simulink model "Punto1_522"  (R2019a)
settings: Solver=VariableStepAuto  StartTime=0.0  StopTime=3  MaxStep=1e-4  RelTol=1e-3
values from neighbouring files (symbols this model uses):
  alfa_cu = 3.9 * 10^(-3)    (= 0.0039)    [Datos.m]
  bl = 0    [Datos.m]
  bm = 1.5 * 10^(-5)    (= 1.5e-05)    [Datos.m]
  Cts = 0.818    [Datos.m]
  Id0 = 0    [Datos.m]    (also in punto6plot.m = 0.5)
  Jl = 0.2520    (= 0.252)    [Datos.m]
  Jm = 3.1 * 10^(-6)    (= 3.1e-06)    [Datos.m]
  Ki0 = 5000*Lls    (= 4)    [Datos.m]
  Kid = 5000*Ld    (= 33)    [Datos.m]
  Kiq = 5000*Lq    (= 29)    [Datos.m]
  lambda_m_r = 0.01546    [Datos.m]
  Ld = 6.6e-3    (= 0.0066)    [Datos.m]
  Lq = 5.8e-3    (= 0.0058)    [Datos.m]
  Pp = 3    [Datos.m]
  r = 314.3008    [Datos.m]
  Rts_amb = 146.7    [Datos.m]
undefined symbols (not defined in the file or in its folder): magnitude
settings Model: Creator=renzo  LastModifiedBy=renzo

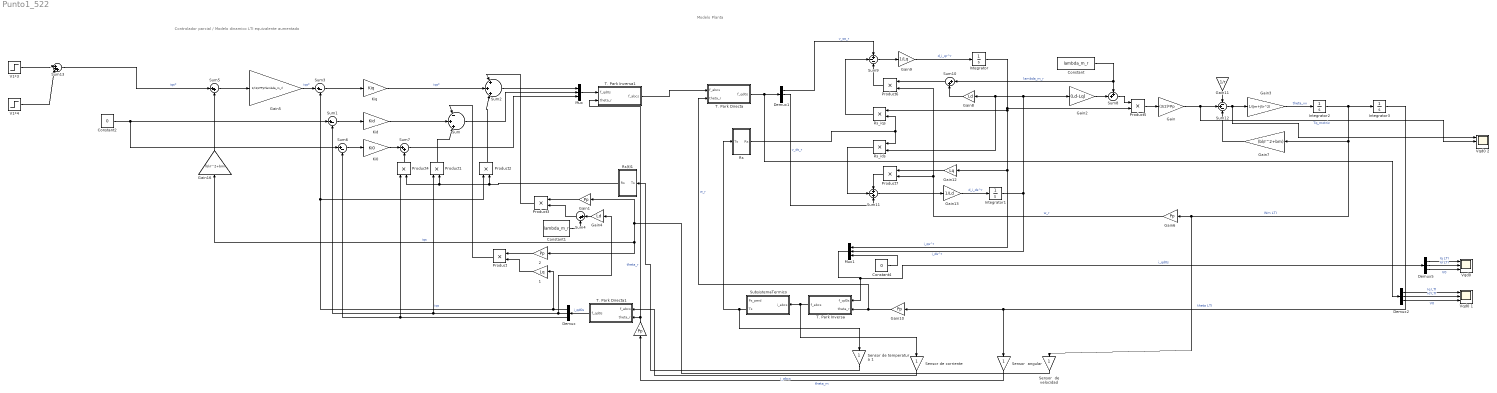
== system Punto1_522 ==
  note: Controlador parcial / Modelo dinamico LTI equivalente aumentado
  note: Modelo Planta
  " " : Gain  Gain=Pp
  " 1" : Gain  Gain=Lq
  " 2" : Gain  Gain=Pp
  Constant : Constant  Value=lambda_m_r
  Constant1 : Constant  Value=lambda_m_r
  Constant2 : Constant  Value=0
  Constant4 : Constant  Value=0
  Demux{,1..2,5} (4 alike) : Demux  Outputs=3
  Gain : Gain  Gain=(3/2)*Pp
  Gain1 : Gain  Gain=Pp
  Gain10 : Gain  Gain=Pp
  Gain11 : Gain  Gain=1/r
  Gain12 : Gain  Gain=Lq
  Gain13 : Gain  Gain=1/Ld
  Gain16 : Gain  Gain=(bl/r^2+bm)
  Gain2 : Gain  Gain=(Ld-Lq)
  Gain3 : Gain  Gain=1/(Jm+Jl/r^2)
  Gain4 : Gain  Gain=Ld
  Gain5 : Gain  Gain=1/(3/2*Pp*lambda_m_r)
  Gain6 : Gain  Gain=Pp
  Gain7 : Gain  Gain=(bl/r^2+bm)
  Gain8 : Gain  Gain=Ld
  Gain9 : Gain  Gain=1/Lq
  Integrator : Integrator
  Integrator1 : Integrator  InitialCondition=Id0
  Integrator2 : Integrator
  Integrator3 : Integrator
  Ki0 : Gain  Gain=Ki0
  Kid : Gain  Gain=Kid
  Kiq : Gain  Gain=Kiq
  Mux : Mux  Inputs=3
  Mux1 : Mux  Inputs=3
  Product{,1..7} (8 alike) : Product
  Rs : Subsystem
  Rs(t)1 : Subsystem
  Rs_ids : Product
  Rs_iqs : Product
  Sensor  angular : Gain
  Sensor  de velocidad : Gain
  "Sensor de corriente " : Gain
  Sensor de temperatura 1 : Gain
  SubsistemaTermico : Subsystem
  Sum : Sum  Inputs=|-|+|+|
  Sum1 : Sum  Inputs=|+-
  Sum{4..5,7,10} (4 alike) : Sum  Inputs=|++
  Sum11 : Sum  Inputs=+-+
  Sum12 : Sum  Inputs=-+-
  Sum13 : Sum  Inputs=|+++
  Sum2 : Sum  Inputs=|+|+|+|
  Sum3 : Sum  Inputs=|+-
  Sum6 : Sum  Inputs=|+-
  Sum8 : Sum  Inputs=++|
  Sum9 : Sum  Inputs=+--
  T. Park Directa : Subsystem
  T. Park Directa1 : Subsystem
  T. Park Inversa : Subsystem
  T. Park Inversa1 : Subsystem
  V1*3 : Step  Time=0.1  After=0.1  SampleTime=0
  V1*4 : Step  Time=0.2  After=-0.1  SampleTime=0
  "Vqd0 " : Scope  NumInputPorts=3
  Vqd0 1 : Scope  NumInputPorts=3
  Vqd0 2 : Scope  NumInputPorts=3
  wires:
  Gain16/1 -> Sum5/2
  Sum1/1 -> Kid/1
  Gain5/1 -> Sum3/1  "iqs*"
  Constant2/1 -> Sum6/1, Sum1/1
  Sum7/1 -> Mux/3
  Demux/1 -> " 1"/1, Sum3/2, Product2/1  "iqs"
  Sum4/1 -> Product3/2
  Sensor de temperatura 1/1 -> Rs(t)1/1(Ts)
  Ki0/1 -> Sum7/1
  Constant1/1 -> Sum4/2
  Sum6/1 -> Ki0/1
  Product4/1 -> Sum7/2
  Product3/1 -> Sum2/1
  Demux/3 -> Product4/1, Sum6/2
  Sum3/1 -> Kiq/1
  Rs(t)1/1(Rs) -> Product4/2, Product1/2, Product2/2
  Sum5/1 -> Gain5/1
  " 2"/1 -> Product/1
  " 1"/1 -> Product/2
  Kiq/1 -> Sum2/2  "iqs*"
  Gain1/1 -> Product3/1
  Sum/1 -> Mux/2
  Gain4/1 -> Sum4/1
  Product1/1 -> Sum/3
  Sum2/1 -> Mux/1
  Product/1 -> Sum/1
  Sensor  de velocidad/1 -> Gain16/1, " 2"/1, Gain1/1  "iqs"
  Mux/1 -> T. Park Inversa1/1(f_qd0s)
  " "/1 -> T. Park Inversa1/2(theta_r), T. Park Directa1/2(theta_r)  "theta_r"
  Kid/1 -> Sum/2
  Sensor  angular/1 -> " "/1  "theta_m"
  "Sensor de corriente "/1 -> T. Park Directa1/1(f_abcs)  "i_abcs"
  T. Park Directa1/1(f_qd0s) -> Demux/1  "i_qd0s"
  Product2/1 -> Sum2/3
  T. Park Inversa1/1(f_abcs) -> T. Park Directa/1(f_abcs)
  Demux/2 -> Gain4/1, Sum1/2, Product1/1
  Sum8/1 -> Product5/1
  T. Park Directa/1(f_qd0s) -> Demux2/1, Demux1/1
  Gain13/1 -> Integrator1/1  "d_i_ds^r"
  Rs_iqs/1 -> Sum9/2
  Gain2/1 -> Sum8/2
  T. Park Inversa/1(f_abcs) -> "Sensor de corriente "/1, SubsistemaTermico/1(i_abcs)
  Gain8/1 -> Sum10/2
  Product7/1 -> Sum11/1
  Sum10/1 -> Product6/1
  Gain7/1 -> Sum12/3
  Gain/1 -> Vqd0 2/2, Sum12/2  "Tq_motriz"
  Integrator3/1 -> Sensor  angular/1, Gain10/1  "theta LTI"
  Sum12/1 -> Vqd0 2/1, Gain3/1
  Rs_ids/1 -> Sum11/2
  Gain10/1 -> T. Park Directa/2(theta_r), T. Park Inversa/2(theta_r)  "w_r"
  Rs/1(Rs) -> Rs_ids/1, Rs_iqs/2
  Constant4/1 -> Mux1/3
  SubsistemaTermico/2(Ts) -> Sensor de temperatura 1/1, Rs/1(Ts)
  Mux1/1 -> Demux5/1, T. Park Inversa/1(f_qd0s)  "i_qd0s"
  Gain3/1 -> Integrator2/1  "theta_vv"
  Integrator/1 -> Product5/2, Mux1/1, Gain12/1, Rs_iqs/1  "i_qs^r"
  Sum11/1 -> Gain13/1
  Product5/1 -> Gain/1
  Integrator1/1 -> Gain8/1, Rs_ids/2, Gain2/1, Mux1/2  "i_ds^r"
  Gain9/1 -> Integrator/1  "d_i_qr^r"
  Integrator2/1 -> Sensor  de velocidad/1, Gain6/1, Gain7/1, Integrator3/1  "Wm LTI"
  Product6/1 -> Sum9/3
  Gain6/1 -> Product6/2, Product7/2  "w_r"
  Demux1/1 -> Sum9/1  "v_qs_r"
  Demux1/2 -> Sum11/3  "v_ds_r"
  Gain11/1 -> Sum12/1
  Sum9/1 -> Gain9/1
  Constant/1 -> Sum8/1, Sum10/1  "lambda_m_r"
  Gain12/1 -> Product7/1
  Demux5/1 -> "Vqd0 "/1  "Iq LTI"
  Demux5/2 -> "Vqd0 "/2  "Id LTI"
  Demux5/3 -> "Vqd0 "/3  "V0"
  Demux2/1 -> Vqd0 1/1  "Iq LTI"
  Demux2/2 -> Vqd0 1/2  "Id LTI"
  Demux2/3 -> Vqd0 1/3  "V0"
  V1*4/1 -> Sum13/2
  Sum13/1 -> Sum5/1  "iqs*"
  V1*3/1 -> Sum13/1

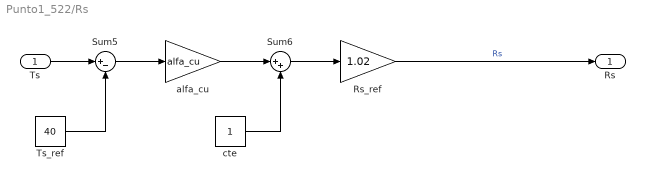
== system Punto1_522/Rs ==
  Ts : Inport
  Rs_ref : Gain  Gain=1.02
  Sum5 : Sum  Inputs=|+-
  Sum6 : Sum  Inputs=|++
  Ts_ref : Constant  Value=40
  alfa_cu : Gain  Gain=alfa_cu
  cte : Constant
  Rs : Outport
  wires:
  Ts_ref/1 -> Sum5/2
  Sum5/1 -> alfa_cu/1
  Sum6/1 -> Rs_ref/1
  Ts/1 -> Sum5/1
  alfa_cu/1 -> Sum6/1
  cte/1 -> Sum6/2
  Rs_ref/1 -> Rs/1  "Rs"

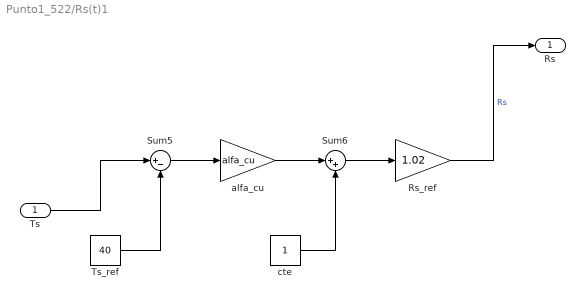
== system Punto1_522/Rs(t)1 ==
  Ts : Inport
  Rs_ref : Gain  Gain=1.02
  Sum5 : Sum  Inputs=|+-
  Sum6 : Sum  Inputs=|++
  Ts_ref : Constant  Value=40
  alfa_cu : Gain  Gain=alfa_cu
  cte : Constant
  Rs : Outport
  wires:
  alfa_cu/1 -> Sum6/1
  Sum6/1 -> Rs_ref/1
  Rs_ref/1 -> Rs/1  "Rs"
  Ts_ref/1 -> Sum5/2
  cte/1 -> Sum6/2
  Ts/1 -> Sum5/1
  Sum5/1 -> alfa_cu/1

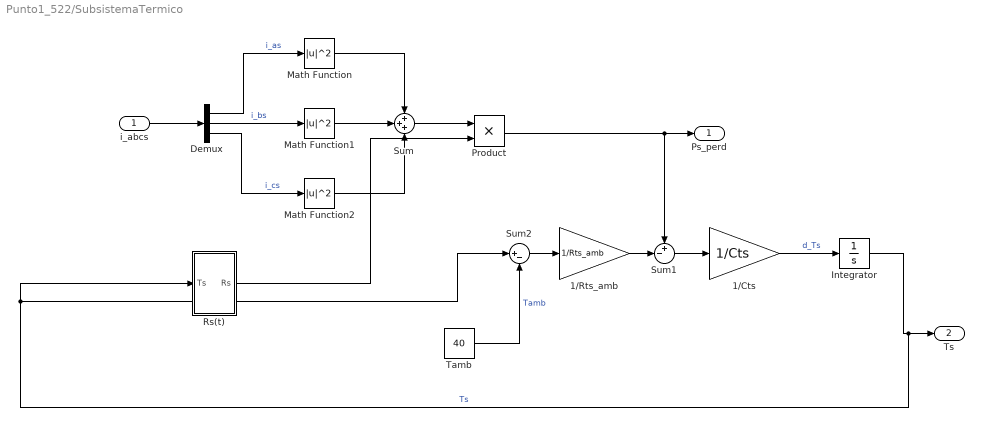
== system Punto1_522/SubsistemaTermico ==
  i_abcs : Inport
  1/Cts : Gain  Gain=1/Cts
  1/Rts_amb : Gain  Gain=1/Rts_amb
  Demux : Demux  Outputs=3
  Integrator : Integrator  InitialCondition=40
  Math Function : Math  Operator=magnitude^2  SaturateOnIntegerOverflow=on
  Math Function1 : Math  Operator=magnitude^2  SaturateOnIntegerOverflow=on
  Math Function2 : Math  Operator=magnitude^2  SaturateOnIntegerOverflow=on
  Product : Product
  Rs(t) : Subsystem
  Sum : Sum  Inputs=3
  Sum1 : Sum  Inputs=+-|
  Sum2 : Sum  Inputs=|+-
  Tamb : Constant  Value=40
  Ps_perd : Outport  VectorParamsAs1DForOutWhenUnconnected=on
  Ts : Outport  Port=2  VectorParamsAs1DForOutWhenUnconnected=on
  wires:
  i_abcs/1 -> Demux/1
  Demux/1 -> Math Function/1  "i_as"
  Demux/2 -> Math Function1/1  "i_bs"
  Demux/3 -> Math Function2/1  "i_cs"
  Math Function1/1 -> Sum/2
  Math Function/1 -> Sum/1
  Math Function2/1 -> Sum/3
  Sum/1 -> Product/1
  Product/1 -> Sum1/1, Ps_perd/1
  Tamb/1 -> Sum2/2  "Tamb"
  Sum2/1 -> 1/Rts_amb/1
  1/Rts_amb/1 -> Sum1/2
  Sum1/1 -> 1/Cts/1
  1/Cts/1 -> Integrator/1  "d_Ts"
  Integrator/1 -> Rs(t)/1(Ts), Sum2/1, Ts/1  "Ts"
  Rs(t)/1(Rs) -> Product/2

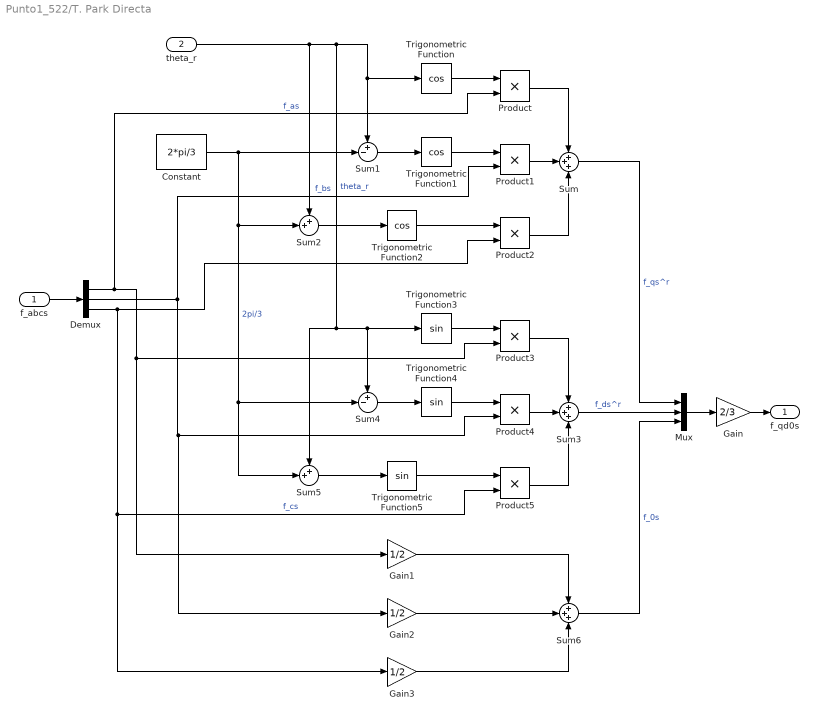
== system Punto1_522/T. Park Directa ==
  f_abcs : Inport
  theta_r : Inport  Port=2
  Constant : Constant  Value=2*pi/3
  Demux : Demux  Outputs=3
  Gain : Gain  Gain=2/3
  Gain1 : Gain  Gain=1/2
  Gain2 : Gain  Gain=1/2
  Gain3 : Gain  Gain=1/2
  Mux : Mux  Inputs=3
  Product{,1..5} (6 alike) : Product
  Sum : Sum  Inputs=3
  Sum1 : Sum  Inputs=+-|
  Sum2 : Sum  Inputs=++|
  Sum3 : Sum  Inputs=3
  Sum4 : Sum  Inputs=+-|
  Sum5 : Sum  Inputs=++|
  Sum6 : Sum  Inputs=3
  Trigonometric Function : Trigonometry  Operator=cos
  Trigonometric Function1 : Trigonometry  Operator=cos
  Trigonometric Function2 : Trigonometry  Operator=cos
  Trigonometric Function3 : Trigonometry
  Trigonometric Function4 : Trigonometry
  Trigonometric Function5 : Trigonometry
  f_qd0s : Outport  VectorParamsAs1DForOutWhenUnconnected=on
  wires:
  Mux/1 -> Gain/1
  f_abcs/1 -> Demux/1
  Demux/1 -> Gain1/1, Product3/2, Product/2  "f_as"
  Demux/2 -> Gain2/1, Product4/2, Product1/2  "f_bs"
  Demux/3 -> Gain3/1, Product5/2, Product2/2  "f_cs"
  Sum/1 -> Mux/1  "f_qs^r"
  Gain/1 -> f_qd0s/1
  Trigonometric Function/1 -> Product/1
  Product/1 -> Sum/1
  Sum1/1 -> Trigonometric Function1/1
  Constant/1 -> Sum5/2, Sum4/2, Sum2/2, Sum1/2  "2pi/3"
  Trigonometric Function1/1 -> Product1/1
  Product1/1 -> Sum/2
  Product2/1 -> Sum/3
  Trigonometric Function2/1 -> Product2/1
  Sum2/1 -> Trigonometric Function2/1
  Product4/1 -> Sum3/2
  Trigonometric Function5/1 -> Product5/1
  Sum5/1 -> Trigonometric Function5/1
  Product5/1 -> Sum3/3
  Product3/1 -> Sum3/1
  Trigonometric Function4/1 -> Product4/1
  Sum4/1 -> Trigonometric Function4/1
  Sum3/1 -> Mux/2  "f_ds^r"
  Trigonometric Function3/1 -> Product3/1
  theta_r/1 -> Sum5/1, Sum4/1, Trigonometric Function3/1, Trigonometric Function/1, Sum1/1, Sum2/1  "theta_r"
  Sum6/1 -> Mux/3  "f_0s"
  Gain3/1 -> Sum6/3
  Gain1/1 -> Sum6/1
  Gain2/1 -> Sum6/2

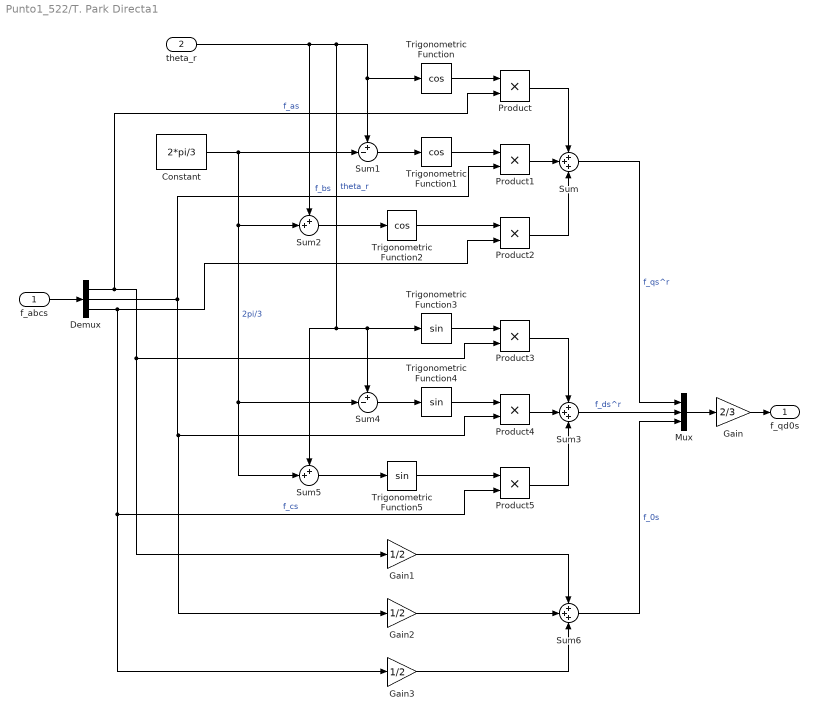
== system Punto1_522/T. Park Directa1 ==
  f_abcs : Inport
  theta_r : Inport  Port=2
  Constant : Constant  Value=2*pi/3
  Demux : Demux  Outputs=3
  Gain : Gain  Gain=2/3
  Gain1 : Gain  Gain=1/2
  Gain2 : Gain  Gain=1/2
  Gain3 : Gain  Gain=1/2
  Mux : Mux  Inputs=3
  Product{,1..5} (6 alike) : Product
  Sum : Sum  Inputs=3
  Sum1 : Sum  Inputs=+-|
  Sum2 : Sum  Inputs=++|
  Sum3 : Sum  Inputs=3
  Sum4 : Sum  Inputs=+-|
  Sum5 : Sum  Inputs=++|
  Sum6 : Sum  Inputs=3
  Trigonometric Function : Trigonometry  Operator=cos
  Trigonometric Function1 : Trigonometry  Operator=cos
  Trigonometric Function2 : Trigonometry  Operator=cos
  Trigonometric Function3 : Trigonometry
  Trigonometric Function4 : Trigonometry
  Trigonometric Function5 : Trigonometry
  f_qd0s : Outport  VectorParamsAs1DForOutWhenUnconnected=on
  wires:
  Mux/1 -> Gain/1
  f_abcs/1 -> Demux/1
  Demux/1 -> Gain1/1, Product3/2, Product/2  "f_as"
  Demux/2 -> Gain2/1, Product4/2, Product1/2  "f_bs"
  Demux/3 -> Gain3/1, Product5/2, Product2/2  "f_cs"
  Sum/1 -> Mux/1  "f_qs^r"
  Gain/1 -> f_qd0s/1
  Trigonometric Function/1 -> Product/1
  Product/1 -> Sum/1
  Sum1/1 -> Trigonometric Function1/1
  Constant/1 -> Sum5/2, Sum4/2, Sum2/2, Sum1/2  "2pi/3"
  Trigonometric Function1/1 -> Product1/1
  Product1/1 -> Sum/2
  Product2/1 -> Sum/3
  Trigonometric Function2/1 -> Product2/1
  Sum2/1 -> Trigonometric Function2/1
  Product4/1 -> Sum3/2
  Trigonometric Function5/1 -> Product5/1
  Sum5/1 -> Trigonometric Function5/1
  Product5/1 -> Sum3/3
  Product3/1 -> Sum3/1
  Trigonometric Function4/1 -> Product4/1
  Sum4/1 -> Trigonometric Function4/1
  Sum3/1 -> Mux/2  "f_ds^r"
  Trigonometric Function3/1 -> Product3/1
  theta_r/1 -> Sum5/1, Sum4/1, Trigonometric Function3/1, Trigonometric Function/1, Sum1/1, Sum2/1  "theta_r"
  Sum6/1 -> Mux/3  "f_0s"
  Gain3/1 -> Sum6/3
  Gain1/1 -> Sum6/1
  Gain2/1 -> Sum6/2

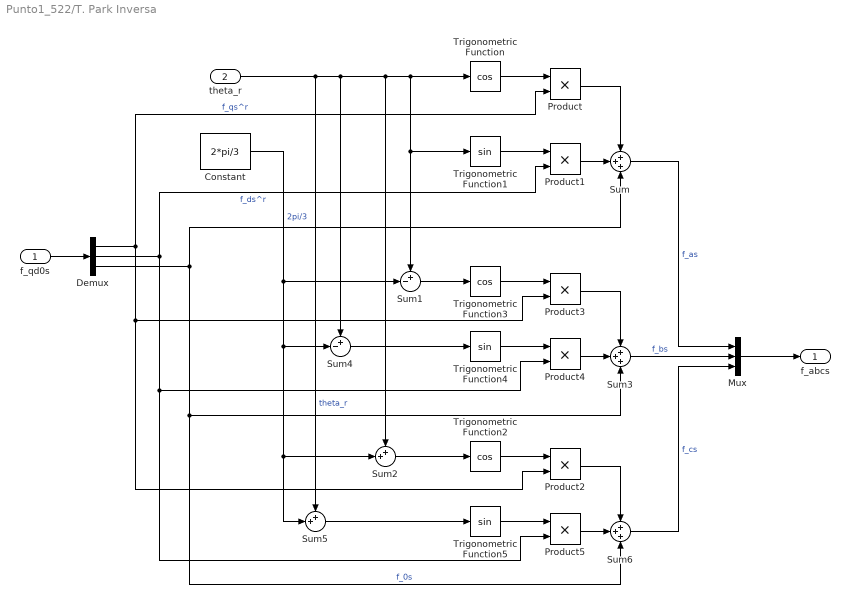
== system Punto1_522/T. Park Inversa ==
  f_qd0s : Inport
  theta_r : Inport  Port=2
  Constant : Constant  Value=2*pi/3
  Demux : Demux  Outputs=3
  Mux : Mux  Inputs=3
  Product{,1..5} (6 alike) : Product
  Sum : Sum  Inputs=3
  Sum1 : Sum  Inputs=+-|
  Sum2 : Sum  Inputs=++|
  Sum3 : Sum  Inputs=3
  Sum4 : Sum  Inputs=+-|
  Sum5 : Sum  Inputs=++|
  Sum6 : Sum  Inputs=3
  Trigonometric Function : Trigonometry  Operator=cos
  Trigonometric Function1 : Trigonometry
  Trigonometric Function2 : Trigonometry  Operator=cos
  Trigonometric Function3 : Trigonometry  Operator=cos
  Trigonometric Function4 : Trigonometry
  Trigonometric Function5 : Trigonometry
  f_abcs : Outport  VectorParamsAs1DForOutWhenUnconnected=on
  wires:
  Trigonometric Function4/1 -> Product4/1
  f_qd0s/1 -> Demux/1
  Trigonometric Function/1 -> Product/1
  Constant/1 -> Sum1/2, Sum4/2, Sum2/2, Sum5/2  "2pi/3"
  Product1/1 -> Sum/2
  Mux/1 -> f_abcs/1
  Sum6/1 -> Mux/3  "f_cs"
  Product/1 -> Sum/1
  theta_r/1 -> Trigonometric Function/1, Trigonometric Function1/1, Sum1/1, Sum2/1, Sum4/1, Sum5/1  "theta_r"
  Product4/1 -> Sum3/2
  Sum3/1 -> Mux/2  "f_bs"
  Trigonometric Function1/1 -> Product1/1
  Sum/1 -> Mux/1  "f_as"
  Trigonometric Function3/1 -> Product3/1
  Product3/1 -> Sum3/1
  Sum4/1 -> Trigonometric Function4/1
  Demux/1 -> Product2/2, Product3/2, Product/2  "f_qs^r"
  Demux/2 -> Product5/2, Product4/2, Product1/2  "f_ds^r"
  Demux/3 -> Sum/3, Sum6/3, Sum3/3  "f_0s"
  Sum1/1 -> Trigonometric Function3/1
  Sum5/1 -> Trigonometric Function5/1
  Trigonometric Function5/1 -> Product5/1
  Trigonometric Function2/1 -> Product2/1
  Product2/1 -> Sum6/1
  Product5/1 -> Sum6/2
  Sum2/1 -> Trigonometric Function2/1

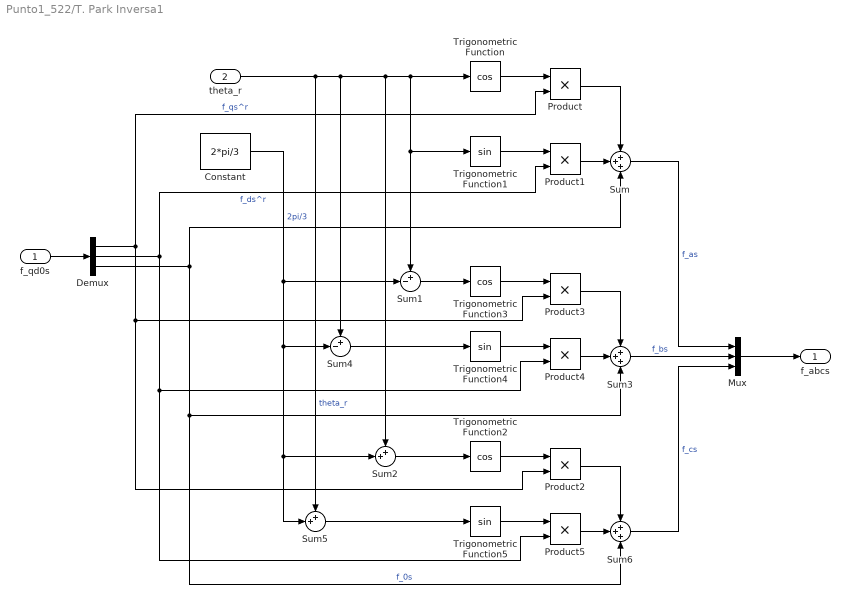
== system Punto1_522/T. Park Inversa1 ==
  f_qd0s : Inport
  theta_r : Inport  Port=2
  Constant : Constant  Value=2*pi/3
  Demux : Demux  Outputs=3
  Mux : Mux  Inputs=3
  Product{,1..5} (6 alike) : Product
  Sum : Sum  Inputs=3
  Sum1 : Sum  Inputs=+-|
  Sum2 : Sum  Inputs=++|
  Sum3 : Sum  Inputs=3
  Sum4 : Sum  Inputs=+-|
  Sum5 : Sum  Inputs=++|
  Sum6 : Sum  Inputs=3
  Trigonometric Function : Trigonometry  Operator=cos
  Trigonometric Function1 : Trigonometry
  Trigonometric Function2 : Trigonometry  Operator=cos
  Trigonometric Function3 : Trigonometry  Operator=cos
  Trigonometric Function4 : Trigonometry
  Trigonometric Function5 : Trigonometry
  f_abcs : Outport  VectorParamsAs1DForOutWhenUnconnected=on
  wires:
  Trigonometric Function4/1 -> Product4/1
  f_qd0s/1 -> Demux/1
  Trigonometric Function/1 -> Product/1
  Constant/1 -> Sum1/2, Sum4/2, Sum2/2, Sum5/2  "2pi/3"
  Product1/1 -> Sum/2
  Mux/1 -> f_abcs/1
  Sum6/1 -> Mux/3  "f_cs"
  Product/1 -> Sum/1
  theta_r/1 -> Trigonometric Function/1, Trigonometric Function1/1, Sum1/1, Sum2/1, Sum4/1, Sum5/1  "theta_r"
  Product4/1 -> Sum3/2
  Sum3/1 -> Mux/2  "f_bs"
  Trigonometric Function1/1 -> Product1/1
  Sum/1 -> Mux/1  "f_as"
  Trigonometric Function3/1 -> Product3/1
  Product3/1 -> Sum3/1
  Sum4/1 -> Trigonometric Function4/1
  Demux/1 -> Product2/2, Product3/2, Product/2  "f_qs^r"
  Demux/2 -> Product5/2, Product4/2, Product1/2  "f_ds^r"
  Demux/3 -> Sum/3, Sum6/3, Sum3/3  "f_0s"
  Sum1/1 -> Trigonometric Function3/1
  Sum5/1 -> Trigonometric Function5/1
  Trigonometric Function5/1 -> Product5/1
  Trigonometric Function2/1 -> Product2/1
  Product2/1 -> Sum6/1
  Product5/1 -> Sum6/2
  Sum2/1 -> Trigonometric Function2/1

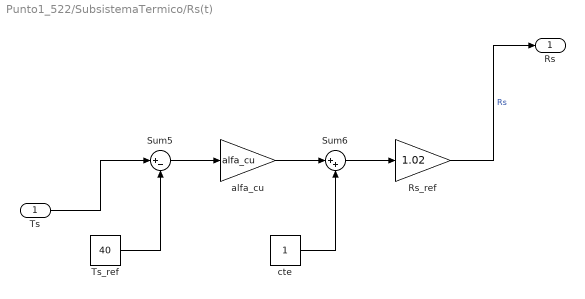
== system Punto1_522/SubsistemaTermico/Rs(t) ==
  Ts : Inport
  Rs_ref : Gain  Gain=1.02
  Sum5 : Sum  Inputs=|+-
  Sum6 : Sum  Inputs=|++
  Ts_ref : Constant  Value=40
  alfa_cu : Gain  Gain=alfa_cu
  cte : Constant
  Rs : Outport
  wires:
  alfa_cu/1 -> Sum6/1
  Sum6/1 -> Rs_ref/1
  Rs_ref/1 -> Rs/1  "Rs"
  Ts_ref/1 -> Sum5/2
  cte/1 -> Sum6/2
  Ts/1 -> Sum5/1
  Sum5/1 -> alfa_cu/1
